simulink model "stepchange_timevarying_change"  (R2022b)
settings: Solver=VariableStepAuto  StartTime=0.0  StopTime=8  RelTol=1e-3
values from neighbouring files (symbols this model uses):
  A = [eye(N),     -LoadZ^-1,   B; zeros(BN,N),  R_l^-1*B',   eye(BN); zeros(1,N),  zeros(1,N),   V_r'*B ]    [stepchange_timevarying_change_initial_document.m]
  A_r = kron(diag(r),eye(N+BN+1))    [stepchange_timevarying_change_initial_document.m]
  alpha_u = [1.1    1.4    1.8    1.1           1.1    1.9    1.9    1.2           1.3    1.4    1.8    0.6           1.8    2.1    1.5    0.9]'    [stepchange_timevarying_change_initial_document.m]
  alpha_V = [0.7    0.6    0.8    0.9           0.7    1.2    0.8    1.24           0.3    0.3    0.0    1.70           1.0    0.5    1.1    1.0]'    [stepchange_timevarying_change_initial_document.m]
  alpha_w = 0.8    [stepchange_timevarying_change_initial_document.m]
  BN = size(Line1,1)/2    [stepchange_timevarying_change_initial_document.m]
  bound_up_vector = zeros(3*N,1)    [stepchange_timevarying_change_initial_document.m]
  changerate = 3    [stepchange_timevarying_change_initial_document.m]
  changetime = 5    [stepchange_timevarying_change_initial_document.m]
  changevariance = 0.1    [stepchange_timevarying_change_initial_document.m]
  constraint_gain = 200    [stepchange_timevarying_change_initial_document.m]
  Dw = 0.01    [stepchange_timevarying_change_initial_document.m]
  epsilon = 2    [stepchange_timevarying_change_initial_document.m]
  F_x = blkdiag(diag(r)*diag(alpha_I)+diag(r)*pr*diag(V_r),diag(r)*diag(alpha_V),F_x_I)    [stepchange_timevarying_change_initial_document.m]
  kappa = 10    [stepchange_timevarying_change_initial_document.m]
  l = 2.5    [stepchange_timevarying_change_initial_document.m]
  lambda_ini = zeros(N*(BN+N+1),1)    [stepchange_timevarying_change_initial_document.m]
  Lap = 1000*(Degree-Adjacent)    [stepchange_timevarying_change_initial_document.m]
  Lap_BN_plus_N = kron(Lap,eye(BN+N+1))    [stepchange_timevarying_change_initial_document.m]
  Lineconstrants = 10*ones(BN,1)    [stepchange_timevarying_change_initial_document.m]
  Lineindex = zeros(BN,4)    [stepchange_timevarying_change_initial_document.m]
  LoadI = [30.0;15.0;30.0;26.0;         18.9;22.8;29.6;32.1;         22.6;27.6;16.5;19.9;         26.5;19.4;22.7;24.9]    [stepchange_timevarying_change_initial_document.m]
  LoadIchange = [30.0;15.0;30.0;26.0;         18.9;22.8;29.6;32.1;         22.6;27.6;16.5;19.9;         26.5;19.4;22.7;24.9]+3*ones(N,1)    [stepchange_timevarying_change_initial_document.m]
  LoadIchangeno = 3    [stepchange_timevarying_change_initial_document.m]
  LoadZ = diag([16.7;50.0;16.7;20.0;              25.0;16.0;14.2;29.4;              18.5;19.6;22.6;25.6;              23.4;26.4;25.2;33.7])    [stepchange_timevarying_change_initial_document.m]
  LoadZchange = diag([16.7;50.0;16.7;20.0;              25.0;16.0;14.2;29.4;              18.5;19.6;22.6;25.6;              23.4;26.4;25.2;33.7])+3*diag(ones(N,1))    [stepchange_timevarying_change_initial_document.m]
  LoadZchangeno = 3    [stepchange_timevarying_change_initial_document.m]
  N = 16    [stepchange_timevarying_change_initial_document.m]
  NCLN = zeros(N,1)    [stepchange_timevarying_change_initial_document.m]
  normal_vector = zeros(3*N,1)    [stepchange_timevarying_change_initial_document.m]
  nu_ini = [-0.00758212493845042	-0.0182492317603708	0.00714905390846842	0.0186908981861182          -0.00758212493845042	-0.0182492317603708	0.00714905390846842	0.0186908981861182          -0.00758212493845042	-0.0182492317603708	0.00714905390846842	0.0186908981861182          -0.00758212493845042	-0.0182492317603708	0.00714905390846842	0.0186908981861182]'    [stepchange_timevarying_change_initial_document.m]
  pr = 0.005    [stepchange_timevarying_change_initial_document.m]
  r = [1.06 1.03 1.05 1.04     1.02 1.03 1.04 1.01     1.03 1.04 1.06 1.07     1.01 1.03 1.04 1.02]    [stepchange_timevarying_change_initial_document.m]
  s_A = zeros(N*(N+BN+1),1)    [stepchange_timevarying_change_initial_document.m]
  theta_ini = zeros(N*(BN+N+1),1)    [stepchange_timevarying_change_initial_document.m]
  u_ini = [378.9289  380.4146  379.7396  379.2243  380.1955  381.1042         379.9247  379.8974  380.0252  380.4045  379.6763  379.8341         380.1194  380.5682  379.3881  379.9696]'    [stepchange_timevarying_change_initial_document.m]
  upsilon_ini = [172.552238898892	172.552238898892	172.552238898892	172.552238898892               172.552238898892	172.552238898892	172.552238898892	172.552238898892               172.552238898892	172.552238898892	172.552238898892	172.552238898892               172.552238898892	172.552238898892	172.552238898892	172.552238898892]'    [stepchange_timevarying_change_initial_document.m]
  V_hat_low = (380-3)*ones(N,1)    [stepchange_timevarying_change_initial_document.m]
  V_hat_up = (380+3)*ones(N,1)    [stepchange_timevarying_change_initial_document.m]
  V_r = [380.16  381.31  380.27  380.13       380.12  381.24  380.15  380.35       380.15  381.13  380.09  380.22       380.19  381.26  380.21  380.19]'    [stepchange_timevarying_change_initial_document.m]
  varepsilon = 50    [stepchange_timevarying_change_initial_document.m]
  x_hat_ini = [14.515064754915	3.95935897697232	32.9787419273847	14.9071228299889             37.6257931691129	61.1095883901259	41.4721611959256	33.6364102939300             44.9867290171943	52.8132621486412	28.1355733315040	33.0707668633162             36.6024320622732	49.3936276267038	2.38033527987224	36.4476162672594             378.638597580330	380.343321138855	379.211948658584	379.000752058610              ...(+639 chars)    [stepchange_timevarying_change_initial_document.m]
undefined symbols (not defined in the file or in its folder): bound_low_vector
libraries: fl_lib x204, nesl_utility x101, simulink x2, spspowerguiLib x1
(part 3 of 3)

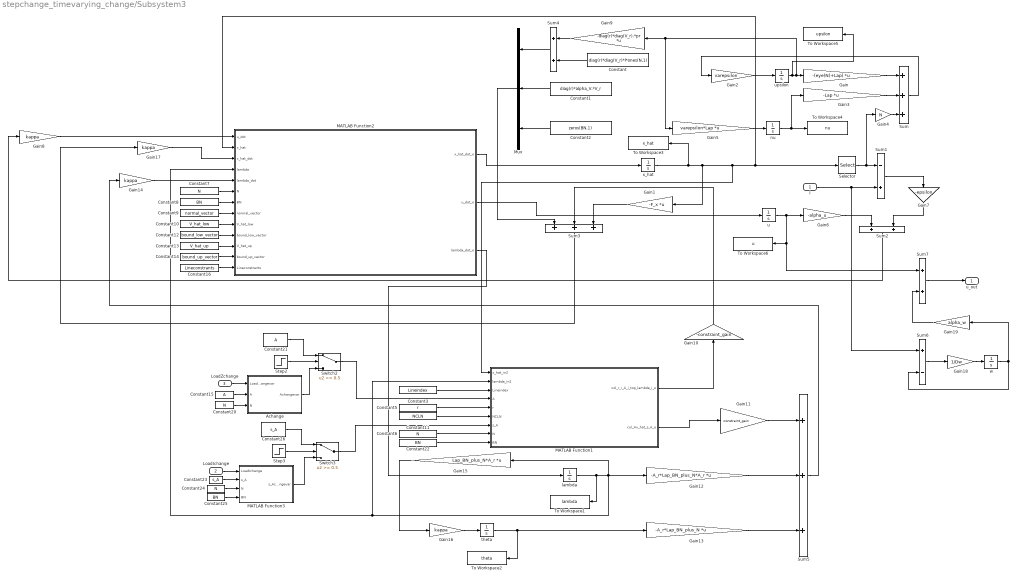
== system stepchange_timevarying_change/Subsystem3 ==
  I : Inport
  LoadIchange : Inport  Port=2
  LoadZchange : Inport  Port=3
  Achange : MATLAB Function  TreatAsAtomicUnit=on
  Constant : Constant  Value=diag(r)*diag(V_r)*l*ones(N,1)
  Constant1 : Constant  Value=diag(r)*alpha_V.*V_r
  Constant10 : Constant  Value=V_hat_low
  Constant11 : Constant  Value=NCLN
  Constant12 : Constant  Value=bound_low_vector
  Constant13 : Constant  Value=V_hat_up
  Constant14 : Constant  Value=bound_up_vector
  Constant15 : Constant  Value=A
  Constant16 : Constant  Value=Lineconstrants
  Constant2 : Constant  Value=zeros(BN,1)
  Constant{6..7,20,24} (4 alike) : Constant  Value=N
  Constant21 : Constant  Value=A
  Constant22 : Constant  Value=BN
  Constant23 : Constant  Value=s_A
  Constant25 : Constant  Value=BN
  Constant26 : Constant  Value=s_A
  Constant3 : Constant  Value=Lineindex
  Constant5 : Constant  Value=r
  Constant8 : Constant  Value=BN
  Constant9 : Constant  Value=normal_vector
  Gain : Gain  Gain=-(eye(N)+Lap)  Multiplication=Matrix(K*u) (u vector)
  Gain1 : Gain  Gain=-F_x  Multiplication=Matrix(K*u) (u vector)
  Gain10 : Gain  Gain=-constraint_gain
  Gain11 : Gain  Gain=constraint_gain
  Gain12 : Gain  Gain=-A_r*Lap_BN_plus_N*A_r  Multiplication=Matrix(K*u) (u vector)
  Gain13 : Gain  Gain=-A_r*Lap_BN_plus_N  Multiplication=Matrix(K*u) (u vector)
  Gain{8,14,16..17} (4 alike) : Gain  Gain=kappa
  Gain15 : Gain  Gain=Lap_BN_plus_N*A_r  Multiplication=Matrix(K*u) (u vector)
  Gain18 : Gain  Gain=1/Dw
  Gain19 : Gain  Gain=alpha_w
  Gain2 : Gain  Gain=varepsilon
  Gain3 : Gain  Gain=-Lap  Multiplication=Matrix(K*u) (u vector)
  Gain4 : Gain  Gain=N
  Gain5 : Gain  Gain=varepsilon*Lap  Multiplication=Matrix(K*u) (u vector)
  Gain6 : Gain  Gain=-alpha_u
  Gain7 : Gain  Gain=-epsilon
  Gain9 : Gain  Gain=-diag(r)*diag(V_r).*pr  Multiplication=Matrix(K*u) (u vector)
  MATLAB Function1 : MATLAB Function  TreatAsAtomicUnit=on
  MATLAB Function2 : MATLAB Function  TreatAsAtomicUnit=on
  MATLAB Function3 : MATLAB Function  TreatAsAtomicUnit=on
  Mux : Mux  Inputs=3
  Selector : Selector  InputPortWidth=52  IndexOptions=Index vector (dialog)  Indices=[1:16]  OutputSizes=1
  Step2 : Step  Time=changetime  Before=1  After=0  SampleTime=0
  Step3 : Step  Time=changetime  Before=1  After=0  SampleTime=0
  Sum : Sum  Inputs=+++
  Sum1 : Sum  Inputs=-+
  Sum2 : Sum
  Sum3 : Sum  Inputs=+++
  Sum4 : Sum
  Sum5 : Sum  Inputs=+++
  Sum6 : Sum  Inputs=+-
  Sum7 : Sum
  Switch2 : Switch  Threshold=0.5  SaturateOnIntegerOverflow=off  InputSameDT=off
  Switch3 : Switch  Threshold=0.5  SaturateOnIntegerOverflow=off  InputSameDT=off
  To Workspace1 : ToWorkspace  VariableName=lambda  SaveFormat=Timeseries  SampleTime=-1
  To Workspace2 : ToWorkspace  VariableName=theta  SaveFormat=Timeseries  SampleTime=-1
  To Workspace3 : ToWorkspace  VariableName=x_hat  SaveFormat=Timeseries  SampleTime=-1
  To Workspace4 : ToWorkspace  VariableName=nu  SaveFormat=Timeseries  SampleTime=-1
  To Workspace5 : ToWorkspace  VariableName=upsilon  SaveFormat=Timeseries  SampleTime=-1
  To Workspace6 : ToWorkspace  VariableName=u  SaveFormat=Timeseries  SampleTime=-1
  lambda : Integrator  InitialCondition=lambda_ini
  nu : Integrator  InitialCondition=nu_ini
  theta : Integrator  InitialCondition=theta_ini
  u : Integrator  InitialCondition=u_ini
  upsilon : Integrator  InitialCondition=upsilon_ini
  w : Integrator  InitialCondition=u_ini
  x_hat : Integrator  InitialCondition=x_hat_ini
  u_out : Outport
  wires:
  MATLAB Function1/2(col_Ax_hat_s_A_o) -> Gain11/1
  MATLAB Function1/1(col_r_i_A_i_top_lambda_i_o) -> Gain10/1
  Constant7/1 -> MATLAB Function2/6(N)
  Constant8/1 -> MATLAB Function2/7(BN)
  Constant9/1 -> MATLAB Function2/8(normal_vector)
  Constant10/1 -> MATLAB Function2/9(V_hat_low)
  Constant12/1 -> MATLAB Function2/10(bound_low_vector)
  Constant13/1 -> MATLAB Function2/11(V_hat_up)
  Constant14/1 -> MATLAB Function2/12(bound_up_vector)
  Constant16/1 -> MATLAB Function2/13(Lineconstrants)
  MATLAB Function2/3(lambda_dot_o) -> lambda/1
  MATLAB Function2/2(u_dot_o) -> u/1
  MATLAB Function2/1(x_hat_dot_o) -> x_hat/1
  Constant6/1 -> MATLAB Function1/8(N)
  Constant5/1 -> MATLAB Function1/5(r)
  Constant11/1 -> MATLAB Function1/6(NCLN)
  Gain14/1 -> MATLAB Function2/5(lambda_dot)
  Gain15/1 -> Gain16/1
  Sum2/1 -> Gain8/1
  Constant2/1 -> Mux/3
  Gain17/1 -> MATLAB Function2/3(x_hat_dot)
  Sum3/1 -> Gain17/1
  Constant3/1 -> MATLAB Function1/3(Lineindex)
  Gain/1 -> Sum/1
  Gain13/1 -> Sum5/3
  Gain9/1 -> Sum4/1
  Sum5/1 -> Gain14/1
  Gain2/1 -> upsilon/1
  Gain8/1 -> MATLAB Function2/1(u_dot)
  Constant1/1 -> Mux/2
  Gain10/1 -> Sum3/2
  Gain3/1 -> Sum/2
  x_hat/1 -> Selector/1, MATLAB Function2/2(x_hat), MATLAB Function1/1(x_hat_in2), Gain1/1, To Workspace3/1
  Gain7/1 -> Sum2/2
  Sum1/1 -> Gain7/1
  Gain1/1 -> Sum3/3
  Mux/1 -> Sum3/1
  Gain11/1 -> Sum5/1
  Sum4/1 -> Mux/1
  theta/1 -> Gain13/1, To Workspace2/1
  upsilon/1 -> Gain/1, Gain9/1, Gain5/1, To Workspace5/1
  Constant22/1 -> MATLAB Function1/9(BN)
  Sum/1 -> Gain2/1
  Gain16/1 -> theta/1
  Gain6/1 -> Sum2/1
  nu/1 -> Gain3/1, To Workspace4/1
  Constant/1 -> Sum4/2
  lambda/1 -> Gain15/1, MATLAB Function1/2(lambda_in2), MATLAB Function2/4(lambda), Gain12/1, To Workspace1/1
  Gain5/1 -> nu/1
  Selector/1 -> Sum1/1, Gain4/1
  I/1 -> Sum1/2, Sum6/1
  u/1 -> Gain6/1, Sum7/1, To Workspace6/1
  Gain4/1 -> Sum/3
  Gain12/1 -> Sum5/2
  Sum6/1 -> Gain18/1
  Gain18/1 -> w/1
  w/1 -> Sum6/2, Gain19/1
  Sum7/1 -> u_out/1
  Gain19/1 -> Sum7/2
  Constant20/1 -> Achange/3(N)
  Achange/1(Achangevar) -> Switch2/3
  LoadZchange/1 -> Achange/1(LoadZchangevar)
  Constant15/1 -> Achange/2(A)
  Step2/1 -> Switch2/2
  Constant21/1 -> Switch2/1
  Switch2/1 -> MATLAB Function1/4(A)
  MATLAB Function3/1(s_Achangevar) -> Switch3/3
  Constant24/1 -> MATLAB Function3/3(N)
  LoadIchange/1 -> MATLAB Function3/1(LoadIchange)
  Constant25/1 -> MATLAB Function3/4(BN)
  Constant23/1 -> MATLAB Function3/2(s_A)
  Step3/1 -> Switch3/2
  Constant26/1 -> Switch3/1
  Switch3/1 -> MATLAB Function1/7(s_A)

== matlab function stepchange_timevarying_change/Subsystem3/Achange ==
  data: LoadZchangevar input; A input; Achangevar output; N input
function Achangevar = fcn(LoadZchangevar,A,N)

A(1:N,N+1:2*N)=zeros(N,N);

Achangevar=A;

Achangevar(1:N,N+1:2*N)=-diag(LoadZchangevar)^-1;

== matlab function stepchange_timevarying_change/Subsystem3/MATLAB Function3 ==
  data: LoadIchange input; s_A input; s_Achangevar output; N input; BN input
function s_Achangevar = fcn(LoadIchange,s_A,N,BN)

for i=1:N

    s_A((i-1)*(N+BN+1)+i,1)=LoadIchange(i);

end

s_Achangevar=s_A;

== matlab function stepchange_timevarying_change/Subsystem3/MATLAB Function1 ==
  data: x_hat_in2 input; col_r_i_A_i_top_lambda_i_o output; lambda_in2 input; Lineindex input; A input; r input; NCLN input; s_A input; N input; BN input; col_Ax_hat_s_A_o output
function [col_r_i_A_i_top_lambda_i_o, col_Ax_hat_s_A_o] = ditributed_calculation(x_hat_in2,lambda_in2,Lineindex, A, r, NCLN, s_A, N, BN)

col_r_i_A_i_top_lambda_i=zeros(52,52)*x_hat_in2;

col_Ax_hat_s_A=zeros(592,1);

A_i_I_l=zeros(592,1);

A_I_l_choose=zeros(20,1);  

        for i=1:N

            A_i_I_l((i-1)*(N+BN+1)+1:i*(N+BN+1))=zeros(N+BN+1,1);

            if NCLN(i,1)~=0

                    check_line_no=find(Lineindex(:,1)==i);

                for j=1:NCLN(i,1)                                          %The numbers of the controlled line of agent i

                    aa=Lineindex(check_line_no(j),4);                                  %choose which line

                    zhong_jian=A_i_I_l((i-1)*(N+BN+1)+1:i*(N+BN+1));
        
                    A_i_I_l((i-1)*(N+BN+1)+1:i*(N+BN+1))=zhong_jian+A(:,2*N+aa)*x_hat_in2(2*N+aa);    %calculate the value of sum B_iI_l_i
                    
                    A_I_l_choose(aa)=r(i)*(A(:,2*N+aa)'*lambda_in2(1+(i-1)*(N+BN+1):i*(N+BN+1)));
        
                end

            end            
            
                col_Ax_hat_s_A(1+(i-1)*(N+BN+1):i*(N+BN+1))=r(i)*(A(:,i)*x_hat_in2(i)+A(:,N+i)*x_hat_in2(i+N)+A_i_I_l((i-1)*(N+BN+1)+1:i*(N+BN+1))-s_A((i-1)*(N+BN+1)+1:i*(N+BN+1)));

                col_r_i_A_i_top_lambda_i(i)=r(i).*A(:,i)'*lambda_in2(1+(i-1)*(N+BN+1):i*(N+BN+1));

                col_r_i_A_i_top_lambda_i(i+N)=r(i).*A(:,N+i)'*lambda_in2(1+(i-1)*(N+BN+1):i*(N+BN+1));

        end

        for i=1:BN

                col_r_i_A_i_top_lambda_i(i+2*N)=A_I_l_choose(i);

        end


        col_r_i_A_i_top_lambda_i_o=col_r_i_A_i_top_lambda_i;

        col_Ax_hat_s_A_o=col_Ax_hat_s_A;

== matlab function stepchange_timevarying_change/Subsystem3/MATLAB Function2 ==
  data: x_hat_dot_o output [..52]; u_dot input size=[16,1]; u_dot_o output size=[16,1]; x_hat input size=[52,1]; x_hat_dot input size=[52,1]; lambda input size=[592,1]; lambda_dot input size=[592,1]; N input; BN input; normal_vector input; V_hat_low input; bound_low_vector input; V_hat_up input; bound_up_vector input; Lineconstrants input; lambda_dot_o output size=[592,1]
function [x_hat_dot_o,u_dot_o,lambda_dot_o] = Projection(u_dot,x_hat,x_hat_dot,lambda,lambda_dot,N,BN,normal_vector,V_hat_low,bound_low_vector,V_hat_up,bound_up_vector,Lineconstrants)

        %---------------------------------projection local constraint cauculation--------------------------------

        projection_judge=zeros(3*N,1);

        projection_vector=zeros(3*N,1);

        for i=1:N                                                                                                       % for all node
            
            projection_judge((i-1)*3+1:3*i)=[u_dot(i);x_hat_dot(i);x_hat_dot(N+i)];

            projection_vector((i-1)*3+1:3*i)=projection_judge((i-1)*3+1:3*i)-projection_judge((i-1)*3+1:3*i)'*normal_vector((i-1)*3+1:3*i)*normal_vector((i-1)*3+1:3*i);
            
            
            if x_hat(N+i)<=V_hat_low(i) && projection_vector(3*i)<0                                                                                 %the projection vector is on the leftside of the feasible set         
                 
                 projection_vector((i-1)*3+1:3*i)=projection_judge((i-1)*3+1:3*i)'*bound_low_vector((i-1)*3+1:3*i)*bound_low_vector((i-1)*3+1:3*i);                           %projection on lower bound
                
             end
             
             if x_hat(N+i)>=V_hat_up(i) && projection_vector(3*i)>0                                                                                     %the projection vector is on the leftside of the feasible set       
                         
                 projection_vector((i-1)*3+1:3*i)=projection_judge((i-1)*3+1:3*i)'*bound_up_vector((i-1)*3+1:3*i)*bound_up_vector((i-1)*3+1:3*i);                                                   %projection on upper bound
                
             end    
             
             u_dot(i,1)=projection_vector((i-1)*3+1);                                                                     % recover the u_g_d dynamic
        
             x_hat_dot(i,1)=projection_vector((i-1)*3+2);                                                                     % recover the I_g_d dynamic
        
             x_hat_dot(N+i,1)=projection_vector((i-1)*3+3);                                                                     % recover the V_g_d dynamic
        
             
        end

        for i=1:BN
        
            if x_hat(2*N+i)>=Lineconstrants(i) &&  x_hat_dot(2*N+i)>0   

                x_hat_dot(2*N+i)=0;

            elseif x_hat(2*N+i)<=-Lineconstrants(i) &&  x_hat_dot(2*N+i)<0

                x_hat_dot(2*N+i)=0;

            end

        end

%---------------------------------projection coupling constraint cauculation--------------------------------


for i=1:N

    if lambda(i*(N+BN+1))<=0 && lambda_dot(i*(N+BN+1))<0

        lambda_dot(i*(N+BN+1))=0;

    end

end

lambda_dot_o=lambda_dot;

u_dot_o=u_dot;

x_hat_dot_o=x_hat_dot;
